simulink model "CusakisME4901"  (R2013a)
settings: Solver=ode3  StartTime=0.0  StopTime=inf  FixedStep=0.01  RelTol=1e-3
InitFcn:
  | start_EEVSCube2
  | 
  | %links masses
  | 
  | m=20;%Kg
  | 
  | l=1;%meter
  | 
  | w=0.08;
  | 
  | I=(1/12)*m*(l^2); %moment of inertia
  | 
  | %estimation error
  | 
  | mn=20+m*0.05;
  | In=I+I*0.1;
  | 
  | %controls
  | 
  | a=0.7; %singularity positive gain
  | 
  | %Chaser
  | mb=1000;%kg
  | lc=2;%meters
  | lb=lc/2;%meter distance 1joint to CM
  | Ib=(1/12)*mb*(lc^2+lc^2);
  | 
  | %Target
  | 
  | mt=750;%kg target mass
  | lt=1;%meter  side lenght
  | It=(1/6)*(lt^2)*mt;
  | 
  | %Target Initial Conitions
  | 
  | x_t=2;
  | y_t=2;
  | theta_t=0.7853;
  | 
  | Init_t=[x_t;y_t;theta_t;0;0;0];
  | Iinv=pinv(eye(3)*It);
StopFcn:
  | figure(1)
  | subplot(2,1,1)
  | hold on
  | plot(time,kinetic,'g')
  | grid on
  | title('Kinetic Energy vs Time')
  | xlabel('Time')
  | ylabel('Kinetic Energy')
  | hold off
  | 
  | subplot(2,1,2)
  | hold on
  | plot(time,power,'g')
  | grid on
  | title('Power Consumption vs Time')
  | xlabel('Time')
  | ylabel('Power')
  | hold off
  | 
  | chasermapping=[-1,1;-1,-1;1,-1;1,1;-1,1];
  | targetmapping=[1.293,2;2,2.707;2.707,2;2,1.293;1.293,2];
  | 
  | figure(3)
  | hold on
  | plot(EEstate(:,1),EEstate(:,2),'g')
  | plot(targetmapping(:,1),targetmapping(:,2),'r')
  | plot(chasermapping(:,1),chasermapping(:,2),'b')
  | grid on
  | title('End Effector Path')
  | xlabel('X Axis (m)')
  | ylabel('Y Axis (m)')
  | hold off
  | 
  | 
  | figure(4)
  | subplot(2,1,1)
  | hold on
  | plot(time,qqd(:,1),'g')
  | plot(time,qqd(:,2),'r')
  | plot(time,qqd(:,3),'b')
  | grid on
  | title('Theta vs Time')
  | xlabel('Time (sec)')
  | ylabel('Theta (rad)')
  | legend( 'Theta1 ' , ' Theta2 ' , ' Theta3')
  | hold off
  | 
  | subplot(2,1,2)
  | hold on
  | plot(time,qqd(:,4),'g')
  | plot(time,qqd(:,5),'r')
  | plot(time,qqd(:,6),'b')
  | grid on
  | legend( 'Omega1 ' , ' Omega2 ', ' Omega3 ' )
  | title('Omega vs Time')
  | xlabel('Time (sec)')
  | ylabel('Omega (rad/s)')
values from neighbouring files (symbols this model uses):
  mesh_A = [mesh_A1 ... (first row only)    [start_EEVSCube2.m]
  mesh_B = [mesh_B1 ... (first row only)    [start_EEVSCube2.m]
undefined symbols (not defined in the file or in its folder): serial
libraries: instrumentlib x5, simulink x3, vrlib x2, dspinverses x1, aerolibanimutils x1
(part 2 of 4)

== matlab function CusakisME4901/Dynamics Block/C Matrix ==
  data: qqd input; C output; mn parameter; l parameter; q_dot output
function [C,q_dot] = fcn(qqd,mn,l)
q=[qqd(7); qqd(8); qqd(9)];
q_dot=[qqd(4); qqd(5); qqd(6)];
C=[                                                                                                                                                                                                                                                                                                                                                                                                                                                                                                                                                  (mn*abs(l)^2*(2*sin(conj(q(1))) + sin(conj(q(1)) + conj(q(2)) + conj(q(3))) + 2*sin(conj(q(1)) + conj(q(2))))*(cos(q(1) + q(2) + q(3))*(q_dot(1) + q_dot(2) + q_dot(3)) + 2*cos(q(1) + q(2))*(q_dot(1) + q_dot(2)) + 2*q_dot(1)*cos(q(1))))/8 - (mn*abs(l)^2*(2*cos(conj(q(1))) + cos(conj(q(1)) + conj(q(2)) + conj(q(3))) + 2*cos(conj(q(1)) + conj(q(2))))*(sin(q(1) + q(2) + q(3))*(q_dot(1) + q_dot(2) + q_dot(3)) + 2*sin(q(1) + q(2))*(q_dot(1) + q_dot(2)) + 2*q_dot(1)*sin(q(1))))/8 + (mn*abs(l)^2*(cos(q(1) + q(2))*(q_dot(1) + q_dot(2)) + 2*q_dot(1)*cos(q(1)))*(2*sin(conj(q(1))) + sin(conj(q(1)) + conj(q(2)))))/8 - (mn*abs(l)^2*(2*cos(conj(q(1))) + cos(conj(q(1)) + conj(q(2))))*(sin(q(1) + q(2))*(q_dot(1) + q_dot(2)) + 2*q_dot(1)*sin(q(1))))/8 - (mn*abs(l)^2*(cos(q(1) + q(2)) + 2*cos(q(1)))*(2*sin(conj(q(1)))*conj(q_dot(1)) + sin(conj(q(1)) + conj(q(2)))*(conj(q_dot(1)) + conj(q_dot(2)))))/8 + (mn*abs(l)^2*(sin(q(1) + q(2)) + 2*sin(q(1)))*(2*cos(conj(q(1)))*conj(q_dot(1)) + cos(conj(q(1)) + conj(q(2)))*(conj(q_dot(1)) + conj(q_dot(2)))))/8 + (mn*abs(l)^2*(2*cos(conj(q(1)))*conj(q_dot(1)) + cos(conj(q(1)) + conj(q(2)) + conj(q(3)))*(conj(q_dot(1)) + conj(q_dot(2)) + conj(q_dot(3))) + 2*cos(conj(q(1)) + conj(q(2)))*(conj(q_dot(1)) + conj(q_dot(2))))*(sin(q(1) + q(2) + q(3)) + 2*sin(q(1) + q(2)) + 2*sin(q(1))))/8 - (mn*abs(l)^2*(2*sin(conj(q(1)))*conj(q_dot(1)) + sin(conj(q(1)) + conj(q(2)) + conj(q(3)))*(conj(q_dot(1)) + conj(q_dot(2)) + conj(q_dot(3))) + 2*sin(conj(q(1)) + conj(q(2)))*(conj(q_dot(1)) + conj(q_dot(2))))*(cos(q(1) + q(2) + q(3)) + 2*cos(q(1) + q(2)) + 2*cos(q(1))))/8 - (mn*q_dot(1)*cos(conj(q(1)))*abs(l)^2*sin(q(1)))/8 + (mn*q_dot(1)*sin(conj(q(1)))*abs(l)^2*cos(q(1)))/8 + (mn*cos(conj(q(1)))*abs(l)^2*conj(q_dot(1))*sin(q(1)))/8 - (mn*sin(conj(q(1)))*abs(l)^2*cos(q(1))*conj(q_dot(1)))/8,                                                                                                                                                                                                                                     (mn*sin(conj(q(1)) - q(2) - q(3) - q(1))*abs(l)^2)/2 + (3*mn*sin(conj(q(1)) - q(2) - q(1))*abs(l)^2)/4 + (mn*abs(l)^2*sin(conj(q(1)) - q(2) - q(3) - q(1) + conj(q(2)))*(q_dot(1) + q_dot(2) + q_dot(3) - conj(q_dot(1)) - conj(q_dot(2))))/4 + (mn*sin(conj(q(1)) - q(2) - q(3) - q(1) + conj(q(2)) + conj(q(3)))*abs(l)^2*(q_dot(1) + q_dot(2) + q_dot(3) - conj(q_dot(1)) - conj(q_dot(2)) - conj(q_dot(3))))/8 - (mn*sin(q(1) + q(2))*abs(l)^2*(2*cos(conj(q(1))) + cos(conj(q(1)) + conj(q(2)))))/8 + (mn*cos(q(1) + q(2))*abs(l)^2*(2*sin(conj(q(1))) + sin(conj(q(1)) + conj(q(2)))))/8 - (mn*abs(l)^2*(sin(conj(q(1)) + conj(q(2)) + conj(q(3))) + 2*sin(conj(q(1)) + conj(q(2))))*(cos(q(1) + q(2) + q(3)) + 2*cos(q(1) + q(2)) + 2*cos(q(1))))/8 + (mn*abs(l)^2*(cos(conj(q(1)) + conj(q(2)) + conj(q(3))) + 2*cos(conj(q(1)) + conj(q(2))))*(sin(q(1) + q(2) + q(3)) + 2*sin(q(1) + q(2)) + 2*sin(q(1))))/8 - (mn*abs(l)^2*sin(conj(q(1)) - q(2) - q(1) + conj(q(2)) + conj(q(3)))*(conj(q_dot(1)) - q_dot(2) - q_dot(1) + conj(q_dot(2)) + conj(q_dot(3))))/4 - (mn*abs(l)^2*(sin(q(1) + q(2) + q(3)) + 2*sin(q(1) + q(2)))*(2*cos(conj(q(1))) + cos(conj(q(1)) + conj(q(2)) + conj(q(3))) + 2*cos(conj(q(1)) + conj(q(2)))))/8 + (mn*abs(l)^2*(cos(q(1) + q(2) + q(3)) + 2*cos(q(1) + q(2)))*(2*sin(conj(q(1))) + sin(conj(q(1)) + conj(q(2)) + conj(q(3))) + 2*sin(conj(q(1)) + conj(q(2)))))/8 - (mn*sin(conj(q(1)) + conj(q(2)))*abs(l)^2*(cos(q(1) + q(2)) + 2*cos(q(1))))/8 + (3*mn*sin(conj(q(1)) - q(2) - q(1))*abs(l)^2*(q_dot(1) + q_dot(2) - conj(q_dot(1))))/4 + (mn*cos(conj(q(1)) + conj(q(2)))*abs(l)^2*(sin(q(1) + q(2)) + 2*sin(q(1))))/8 + (5*mn*sin(conj(q(1)) - q(2) - q(1) + conj(q(2)))*abs(l)^2*(q_dot(1) + q_dot(2) - conj(q_dot(1)) - conj(q_dot(2))))/8 + (mn*sin(conj(q(1)) - q(2) - q(3) - q(1))*abs(l)^2*(q_dot(1) + q_dot(2) + q_dot(3) - conj(q_dot(1))))/4, (mn*sin(conj(q(1)) - q(2) - q(3) - q(1))*abs(l)^2)/4 + (mn*abs(l)^2*(2*sin(conj(q(1)) - q(2) - q(3) - q(1)) + 2*sin(conj(q(1)) - q(2) - q(3) - q(1) + conj(q(2)))))/8 + (mn*abs(l)^2*(2*sin(conj(q(1)) - q(2) - q(3) - q(1))*(q_dot(1) + q_dot(2) + q_dot(3) - conj(q_dot(1))) + 2*sin(conj(q(1)) - q(2) - q(3) - q(1) + conj(q(2)))*(q_dot(1) + q_dot(2) + q_dot(3) - conj(q_dot(1)) - conj(q_dot(2))) + sin(conj(q(1)) - q(2) - q(3) - q(1) + conj(q(2)) + conj(q(3)))*(q_dot(1) + q_dot(2) + q_dot(3) - conj(q_dot(1)) - conj(q_dot(2)) - conj(q_dot(3)))))/8 + (mn*abs(l)^2*sin(conj(q(1)) - q(2) - q(3) - q(1) + conj(q(2))))/4 - (mn*abs(l)^2*sin(conj(q(1)) - q(2) - q(1) + conj(q(2)) + conj(q(3))))/4 + (mn*cos(conj(q(1)) + conj(q(2)) + conj(q(3)))*abs(l)^2*(sin(q(1) + q(2) + q(3)) + 2*sin(q(1) + q(2)) + 2*sin(q(1))))/8 - (mn*sin(q(1) + q(2) + q(3))*abs(l)^2*(2*cos(conj(q(1))) + cos(conj(q(1)) + conj(q(2)) + conj(q(3))) + 2*cos(conj(q(1)) + conj(q(2)))))/8 + (mn*cos(q(1) + q(2) + q(3))*abs(l)^2*(2*sin(conj(q(1))) + sin(conj(q(1)) + conj(q(2)) + conj(q(3))) + 2*sin(conj(q(1)) + conj(q(2)))))/8 - (mn*sin(conj(q(1)) + conj(q(2)) + conj(q(3)))*abs(l)^2*(cos(q(1) + q(2) + q(3)) + 2*cos(q(1) + q(2)) + 2*cos(q(1))))/8;
 (mn*sin(conj(q(1)) - q(2) - q(3) - q(1))*abs(l)^2)/2 + (3*mn*sin(conj(q(1)) - q(2) - q(1))*abs(l)^2)/4 - (mn*abs(l)^2*(cos(conj(q(1)) + conj(q(2)) + conj(q(3))) + 2*cos(conj(q(1)) + conj(q(2))))*(sin(q(1) + q(2) + q(3))*(q_dot(1) + q_dot(2) + q_dot(3)) + 2*sin(q(1) + q(2))*(q_dot(1) + q_dot(2)) + 2*q_dot(1)*sin(q(1))))/8 - (mn*sin(q(1) + q(2))*abs(l)^2*(2*cos(conj(q(1))) + cos(conj(q(1)) + conj(q(2)))))/8 + (mn*cos(q(1) + q(2))*abs(l)^2*(2*sin(conj(q(1))) + sin(conj(q(1)) + conj(q(2)))))/8 - (mn*abs(l)^2*(sin(conj(q(1)) + conj(q(2)) + conj(q(3))) + 2*sin(conj(q(1)) + conj(q(2))))*(cos(q(1) + q(2) + q(3)) + 2*cos(q(1) + q(2)) + 2*cos(q(1))))/8 + (mn*abs(l)^2*(cos(conj(q(1)) + conj(q(2)) + conj(q(3))) + 2*cos(conj(q(1)) + conj(q(2))))*(sin(q(1) + q(2) + q(3)) + 2*sin(q(1) + q(2)) + 2*sin(q(1))))/8 - (mn*abs(l)^2*(sin(conj(q(1)) + conj(q(2)) + conj(q(3)))*(conj(q_dot(1)) + conj(q_dot(2)) + conj(q_dot(3))) + 2*sin(conj(q(1)) + conj(q(2)))*(conj(q_dot(1)) + conj(q_dot(2))))*(cos(q(1) + q(2) + q(3)) + 2*cos(q(1) + q(2)) + 2*cos(q(1))))/8 + (mn*abs(l)^2*(cos(conj(q(1)) + conj(q(2)) + conj(q(3)))*(conj(q_dot(1)) + conj(q_dot(2)) + conj(q_dot(3))) + 2*cos(conj(q(1)) + conj(q(2)))*(conj(q_dot(1)) + conj(q_dot(2))))*(sin(q(1) + q(2) + q(3)) + 2*sin(q(1) + q(2)) + 2*sin(q(1))))/8 - (mn*abs(l)^2*(sin(q(1) + q(2) + q(3)) + 2*sin(q(1) + q(2)))*(2*cos(conj(q(1))) + cos(conj(q(1)) + conj(q(2)) + conj(q(3))) + 2*cos(conj(q(1)) + conj(q(2)))))/8 + (mn*abs(l)^2*(cos(q(1) + q(2) + q(3)) + 2*cos(q(1) + q(2)))*(2*sin(conj(q(1))) + sin(conj(q(1)) + conj(q(2)) + conj(q(3))) + 2*sin(conj(q(1)) + conj(q(2)))))/8 - (mn*sin(conj(q(1)) + conj(q(2)))*abs(l)^2*(cos(q(1) + q(2)) + 2*cos(q(1))))/8 + (mn*cos(conj(q(1)) + conj(q(2)))*abs(l)^2*(sin(q(1) + q(2)) + 2*sin(q(1))))/8 + (mn*sin(conj(q(1)) + conj(q(2)))*abs(l)^2*(cos(q(1) + q(2))*(q_dot(1) + q_dot(2)) + 2*q_dot(1)*cos(q(1))))/8 - (mn*cos(conj(q(1)) + conj(q(2)))*abs(l)^2*(sin(q(1) + q(2))*(q_dot(1) + q_dot(2)) + 2*q_dot(1)*sin(q(1))))/8 + (mn*abs(l)^2*(sin(conj(q(1)) + conj(q(2)) + conj(q(3))) + 2*sin(conj(q(1)) + conj(q(2))))*(cos(q(1) + q(2) + q(3))*(q_dot(1) + q_dot(2) + q_dot(3)) + 2*cos(q(1) + q(2))*(q_dot(1) + q_dot(2)) + 2*q_dot(1)*cos(q(1))))/8 - (mn*sin(conj(q(1)) + conj(q(2)))*abs(l)^2*(conj(q_dot(1)) + conj(q_dot(2)))*(cos(q(1) + q(2)) + 2*cos(q(1))))/8 + (mn*cos(conj(q(1)) + conj(q(2)))*abs(l)^2*(conj(q_dot(1)) + conj(q_dot(2)))*(sin(q(1) + q(2)) + 2*sin(q(1))))/8, (mn*sin(conj(q(1)) + conj(q(2)))*cos(q(1) + q(2))*abs(l)^2)/4 - (mn*cos(conj(q(1)) + conj(q(2)))*sin(q(1) + q(2))*abs(l)^2)/4 - (mn*abs(l)^2*(sin(conj(q(1)) + conj(q(2)) + conj(q(3))) + 2*sin(conj(q(1)) + conj(q(2))))*(cos(q(1) + q(2) + q(3)) + 2*cos(q(1) + q(2)) + 2*cos(q(1))))/4 + (mn*abs(l)^2*(cos(conj(q(1)) + conj(q(2)) + conj(q(3))) + 2*cos(conj(q(1)) + conj(q(2))))*(sin(q(1) + q(2) + q(3)) + 2*sin(q(1) + q(2)) + 2*sin(q(1))))/4 - (mn*abs(l)^2*(cos(q(1) + q(2) + q(3)) + 2*cos(q(1) + q(2)))*(sin(conj(q(1)) + conj(q(2)) + conj(q(3)))*(conj(q_dot(1)) + conj(q_dot(2)) + conj(q_dot(3))) + 2*sin(conj(q(1)) + conj(q(2)))*(conj(q_dot(1)) + conj(q_dot(2)))))/8 + (mn*abs(l)^2*(sin(q(1) + q(2) + q(3)) + 2*sin(q(1) + q(2)))*(cos(conj(q(1)) + conj(q(2)) + conj(q(3)))*(conj(q_dot(1)) + conj(q_dot(2)) + conj(q_dot(3))) + 2*cos(conj(q(1)) + conj(q(2)))*(conj(q_dot(1)) + conj(q_dot(2)))))/8 - (mn*abs(l)^2*(cos(conj(q(1)) + conj(q(2)) + conj(q(3))) + 2*cos(conj(q(1)) + conj(q(2))))*(sin(q(1) + q(2) + q(3))*(q_dot(1) + q_dot(2) + q_dot(3)) + 2*sin(q(1) + q(2))*(q_dot(1) + q_dot(2))))/8 + (mn*abs(l)^2*(sin(conj(q(1)) + conj(q(2)) + conj(q(3))) + 2*sin(conj(q(1)) + conj(q(2))))*(cos(q(1) + q(2) + q(3))*(q_dot(1) + q_dot(2) + q_dot(3)) + 2*cos(q(1) + q(2))*(q_dot(1) + q_dot(2))))/8 - (mn*sin(conj(q(1)) + conj(q(2)))*abs(l)^2*(cos(q(1) + q(2)) + 2*cos(q(1))))/4 + (mn*cos(conj(q(1)) + conj(q(2)))*abs(l)^2*(sin(q(1) + q(2)) + 2*sin(q(1))))/4 - (mn*abs(l)^2*(cos(conj(q(1)) + conj(q(2)) + conj(q(3))) + 2*cos(conj(q(1)) + conj(q(2))))*(sin(q(1) + q(2) + q(3)) + 2*sin(q(1) + q(2))))/4 + (mn*abs(l)^2*(cos(q(1) + q(2) + q(3)) + 2*cos(q(1) + q(2)))*(sin(conj(q(1)) + conj(q(2)) + conj(q(3))) + 2*sin(conj(q(1)) + conj(q(2)))))/4 + (mn*cos(conj(q(1)) + conj(q(2)))*sin(q(1) + q(2))*abs(l)^2*(conj(q_dot(1)) + conj(q_dot(2))))/8 - (mn*sin(conj(q(1)) + conj(q(2)))*cos(q(1) + q(2))*abs(l)^2*(conj(q_dot(1)) + conj(q_dot(2))))/8 - (mn*cos(conj(q(1)) + conj(q(2)))*sin(q(1) + q(2))*abs(l)^2*(q_dot(1) + q_dot(2)))/8 + (mn*sin(conj(q(1)) + conj(q(2)))*cos(q(1) + q(2))*abs(l)^2*(q_dot(1) + q_dot(2)))/8,                                                                                                                                                                                                                                                                                                                       (mn*abs(l)^2*(2*sin(conj(q(1)) - q(2) - q(3) - q(1) + conj(q(2)))*(q_dot(1) + q_dot(2) + q_dot(3) - conj(q_dot(1)) - conj(q_dot(2))) + sin(conj(q(1)) - q(2) - q(3) - q(1) + conj(q(2)) + conj(q(3)))*(q_dot(1) + q_dot(2) + q_dot(3) - conj(q_dot(1)) - conj(q_dot(2)) - conj(q_dot(3)))))/8 + (mn*abs(l)^2*sin(conj(q(1)) - q(2) - q(3) - q(1) + conj(q(2))))/4 + (mn*cos(conj(q(1)) + conj(q(2)) + conj(q(3)))*abs(l)^2*(sin(q(1) + q(2) + q(3)) + 2*sin(q(1) + q(2)) + 2*sin(q(1))))/4 - (mn*sin(q(1) + q(2) + q(3))*abs(l)^2*(cos(conj(q(1)) + conj(q(2)) + conj(q(3))) + 2*cos(conj(q(1)) + conj(q(2)))))/4 + (mn*cos(q(1) + q(2) + q(3))*abs(l)^2*(sin(conj(q(1)) + conj(q(2)) + conj(q(3))) + 2*sin(conj(q(1)) + conj(q(2)))))/4 - (mn*sin(conj(q(1)) + conj(q(2)) + conj(q(3)))*abs(l)^2*(cos(q(1) + q(2) + q(3)) + 2*cos(q(1) + q(2)) + 2*cos(q(1))))/4;
                                                                                                                                                                                                                                                                                                                                                                                                                                                                                                                                                                                                                                                                                                                                                                                                      (mn*sin(conj(q(1)) - q(2) - q(3) - q(1))*abs(l)^2)/4 + (mn*abs(l)^2*(2*sin(conj(q(1)) - q(2) - q(3) - q(1)) + 2*sin(conj(q(1)) - q(2) - q(3) - q(1) + conj(q(2)))))/8 + (mn*abs(l)^2*sin(conj(q(1)) - q(2) - q(3) - q(1) + conj(q(2))))/4 - (mn*abs(l)^2*sin(conj(q(1)) - q(2) - q(1) + conj(q(2)) + conj(q(3))))/4 + (mn*cos(conj(q(1)) + conj(q(2)) + conj(q(3)))*abs(l)^2*(sin(q(1) + q(2) + q(3)) + 2*sin(q(1) + q(2)) + 2*sin(q(1))))/8 - (mn*sin(q(1) + q(2) + q(3))*abs(l)^2*(2*cos(conj(q(1))) + cos(conj(q(1)) + conj(q(2)) + conj(q(3))) + 2*cos(conj(q(1)) + conj(q(2)))))/8 + (mn*cos(q(1) + q(2) + q(3))*abs(l)^2*(2*sin(conj(q(1))) + sin(conj(q(1)) + conj(q(2)) + conj(q(3))) + 2*sin(conj(q(1)) + conj(q(2)))))/8 + (mn*sin(conj(q(1)) + conj(q(2)) + conj(q(3)))*abs(l)^2*(cos(q(1) + q(2) + q(3))*(q_dot(1) + q_dot(2) + q_dot(3)) + 2*cos(q(1) + q(2))*(q_dot(1) + q_dot(2)) + 2*q_dot(1)*cos(q(1))))/8 - (mn*cos(conj(q(1)) + conj(q(2)) + conj(q(3)))*abs(l)^2*(sin(q(1) + q(2) + q(3))*(q_dot(1) + q_dot(2) + q_dot(3)) + 2*sin(q(1) + q(2))*(q_dot(1) + q_dot(2)) + 2*q_dot(1)*sin(q(1))))/8 - (mn*sin(conj(q(1)) + conj(q(2)) + conj(q(3)))*abs(l)^2*(cos(q(1) + q(2) + q(3)) + 2*cos(q(1) + q(2)) + 2*cos(q(1))))/8 - (mn*sin(conj(q(1)) + conj(q(2)) + conj(q(3)))*abs(l)^2*(cos(q(1) + q(2) + q(3)) + 2*cos(q(1) + q(2)) + 2*cos(q(1)))*(conj(q_dot(1)) + conj(q_dot(2)) + conj(q_dot(3))))/8 + (mn*cos(conj(q(1)) + conj(q(2)) + conj(q(3)))*abs(l)^2*(sin(q(1) + q(2) + q(3)) + 2*sin(q(1) + q(2)) + 2*sin(q(1)))*(conj(q_dot(1)) + conj(q_dot(2)) + conj(q_dot(3))))/8,                                                                                                                                                                                                                                                                                                                                                                                                                                                                                                                                                                                                                                                                                                                                                                                                            (mn*abs(l)^2*sin(conj(q(1)) - q(2) - q(3) - q(1) + conj(q(2))))/4 + (mn*cos(conj(q(1)) + conj(q(2)) + conj(q(3)))*abs(l)^2*(sin(q(1) + q(2) + q(3)) + 2*sin(q(1) + q(2)) + 2*sin(q(1))))/4 + (mn*sin(conj(q(1)) + conj(q(2)) + conj(q(3)))*abs(l)^2*(cos(q(1) + q(2) + q(3))*(q_dot(1) + q_dot(2) + q_dot(3)) + 2*cos(q(1) + q(2))*(q_dot(1) + q_dot(2))))/8 - (mn*cos(conj(q(1)) + conj(q(2)) + conj(q(3)))*abs(l)^2*(sin(q(1) + q(2) + q(3))*(q_dot(1) + q_dot(2) + q_dot(3)) + 2*sin(q(1) + q(2))*(q_dot(1) + q_dot(2))))/8 - (mn*sin(q(1) + q(2) + q(3))*abs(l)^2*(cos(conj(q(1)) + conj(q(2)) + conj(q(3))) + 2*cos(conj(q(1)) + conj(q(2)))))/4 + (mn*cos(q(1) + q(2) + q(3))*abs(l)^2*(sin(conj(q(1)) + conj(q(2)) + conj(q(3))) + 2*sin(conj(q(1)) + conj(q(2)))))/4 - (mn*sin(conj(q(1)) + conj(q(2)) + conj(q(3)))*abs(l)^2*(cos(q(1) + q(2) + q(3)) + 2*cos(q(1) + q(2)) + 2*cos(q(1))))/4 - (mn*sin(conj(q(1)) + conj(q(2)) + conj(q(3)))*abs(l)^2*(cos(q(1) + q(2) + q(3)) + 2*cos(q(1) + q(2)))*(conj(q_dot(1)) + conj(q_dot(2)) + conj(q_dot(3))))/8 + (mn*cos(conj(q(1)) + conj(q(2)) + conj(q(3)))*abs(l)^2*(sin(q(1) + q(2) + q(3)) + 2*sin(q(1) + q(2)))*(conj(q_dot(1)) + conj(q_dot(2)) + conj(q_dot(3))))/8,                                                                                                                                                                                                                                                                                                                                                            (mn*sin(conj(q(1)) - q(2) - q(3) - q(1) + conj(q(2)) + conj(q(3)))*abs(l)^2*(q_dot(1) + q_dot(2) + q_dot(3) - conj(q_dot(1)) - conj(q_dot(2)) - conj(q_dot(3))))/8 + (mn*cos(conj(q(1)) + conj(q(2)) + conj(q(3)))*abs(l)^2*(sin(q(1) + q(2) + q(3)) + 2*sin(q(1) + q(2)) + 2*sin(q(1))))/4 + (mn*cos(q(1) + q(2) + q(3))*sin(conj(q(1)) + conj(q(2)) + conj(q(3)))*abs(l)^2)/2 - (mn*sin(q(1) + q(2) + q(3))*cos(conj(q(1)) + conj(q(2)) + conj(q(3)))*abs(l)^2)/2 - (mn*sin(conj(q(1)) + conj(q(2)) + conj(q(3)))*abs(l)^2*(cos(q(1) + q(2) + q(3)) + 2*cos(q(1) + q(2))))/4 + (mn*cos(conj(q(1)) + conj(q(2)) + conj(q(3)))*abs(l)^2*(sin(q(1) + q(2) + q(3)) + 2*sin(q(1) + q(2))))/4 - (mn*sin(conj(q(1)) + conj(q(2)) + conj(q(3)))*abs(l)^2*(cos(q(1) + q(2) + q(3)) + 2*cos(q(1) + q(2)) + 2*cos(q(1))))/4];

== matlab function CusakisME4901/Dynamics Block/G Matrix (set to zero) ==
  data: qqd input; G output; l parameter; m parameter
function G = fcn(qqd,l,m)

q=[qqd(7) qqd(8) qqd(9)];

g=[0 9.81 0]; %gravity acceleration along y


Jp1=[-(l/2)*sin(q(1)) 0 0; (l/2)*cos(q(1)) 0 0; 0 0 0];
Jo1=[0 0 0; 0 0 0; 1 0 0];

Jp2=[-l*sin(q(1))-(l/2)*sin(q(1)+q(2)) -(l/2)*sin(q(1)+q(2)) 0 ;    l*cos(q(1))+(l/2)*cos(q(1)+q(2)) (l/2)*cos(q(1)+q(2)) 0; 0 0 0];
Jo2=[0 0 0; 0 0 0; 1 1 0];

Jp3=[-l*sin(q(1))-l*sin(q(1)+q(2))-(l/2)*sin(q(1)+q(2)+q(3)) -l*sin(q(1)+q(2))-(l/2)*sin(q(1)+q(2)+q(3)) -(l/2)*sin(q(1)+q(2)+q(3)); l*cos(q(1))+(l)*cos(q(1)+q(2))+(l/2)*cos(q(1)+q(2)+q(3)) l*cos(q(1)+q(2))+(l/2)*cos(q(1)+q(2)+q(3)) (l/2)*cos(q(1)+q(2)+q(3)); 0 0 0];
Jo3=[0 0 0; 0 0 0; 1 1 1];

G1=m*(g)*Jp1+m*(g)*Jp2+m*(g)*Jp3;

%G=G1.';

G=[0;0;0];

== matlab function CusakisME4901/Torque Control/C Matrix ==
  data: qqd input; C output; m parameter; l parameter; q_dot output
function [C,q_dot] = fcn(qqd,m,l)
q=[qqd(7); qqd(8); qqd(9)];
q_dot=[qqd(4); qqd(5); qqd(6)];
C=[                                                                                                                                                                                                                                                                                                                                                                                                                                                                                                                                                  (m*abs(l)^2*(2*sin(conj(q(1))) + sin(conj(q(1)) + conj(q(2)) + conj(q(3))) + 2*sin(conj(q(1)) + conj(q(2))))*(cos(q(1) + q(2) + q(3))*(q_dot(1) + q_dot(2) + q_dot(3)) + 2*cos(q(1) + q(2))*(q_dot(1) + q_dot(2)) + 2*q_dot(1)*cos(q(1))))/8 - (m*abs(l)^2*(2*cos(conj(q(1))) + cos(conj(q(1)) + conj(q(2)) + conj(q(3))) + 2*cos(conj(q(1)) + conj(q(2))))*(sin(q(1) + q(2) + q(3))*(q_dot(1) + q_dot(2) + q_dot(3)) + 2*sin(q(1) + q(2))*(q_dot(1) + q_dot(2)) + 2*q_dot(1)*sin(q(1))))/8 + (m*abs(l)^2*(cos(q(1) + q(2))*(q_dot(1) + q_dot(2)) + 2*q_dot(1)*cos(q(1)))*(2*sin(conj(q(1))) + sin(conj(q(1)) + conj(q(2)))))/8 - (m*abs(l)^2*(2*cos(conj(q(1))) + cos(conj(q(1)) + conj(q(2))))*(sin(q(1) + q(2))*(q_dot(1) + q_dot(2)) + 2*q_dot(1)*sin(q(1))))/8 - (m*abs(l)^2*(cos(q(1) + q(2)) + 2*cos(q(1)))*(2*sin(conj(q(1)))*conj(q_dot(1)) + sin(conj(q(1)) + conj(q(2)))*(conj(q_dot(1)) + conj(q_dot(2)))))/8 + (m*abs(l)^2*(sin(q(1) + q(2)) + 2*sin(q(1)))*(2*cos(conj(q(1)))*conj(q_dot(1)) + cos(conj(q(1)) + conj(q(2)))*(conj(q_dot(1)) + conj(q_dot(2)))))/8 + (m*abs(l)^2*(2*cos(conj(q(1)))*conj(q_dot(1)) + cos(conj(q(1)) + conj(q(2)) + conj(q(3)))*(conj(q_dot(1)) + conj(q_dot(2)) + conj(q_dot(3))) + 2*cos(conj(q(1)) + conj(q(2)))*(conj(q_dot(1)) + conj(q_dot(2))))*(sin(q(1) + q(2) + q(3)) + 2*sin(q(1) + q(2)) + 2*sin(q(1))))/8 - (m*abs(l)^2*(2*sin(conj(q(1)))*conj(q_dot(1)) + sin(conj(q(1)) + conj(q(2)) + conj(q(3)))*(conj(q_dot(1)) + conj(q_dot(2)) + conj(q_dot(3))) + 2*sin(conj(q(1)) + conj(q(2)))*(conj(q_dot(1)) + conj(q_dot(2))))*(cos(q(1) + q(2) + q(3)) + 2*cos(q(1) + q(2)) + 2*cos(q(1))))/8 - (m*q_dot(1)*cos(conj(q(1)))*abs(l)^2*sin(q(1)))/8 + (m*q_dot(1)*sin(conj(q(1)))*abs(l)^2*cos(q(1)))/8 + (m*cos(conj(q(1)))*abs(l)^2*conj(q_dot(1))*sin(q(1)))/8 - (m*sin(conj(q(1)))*abs(l)^2*cos(q(1))*conj(q_dot(1)))/8,                                                                                                                                                                                                                                     (m*sin(conj(q(1)) - q(2) - q(3) - q(1))*abs(l)^2)/2 + (3*m*sin(conj(q(1)) - q(2) - q(1))*abs(l)^2)/4 + (m*abs(l)^2*sin(conj(q(1)) - q(2) - q(3) - q(1) + conj(q(2)))*(q_dot(1) + q_dot(2) + q_dot(3) - conj(q_dot(1)) - conj(q_dot(2))))/4 + (m*sin(conj(q(1)) - q(2) - q(3) - q(1) + conj(q(2)) + conj(q(3)))*abs(l)^2*(q_dot(1) + q_dot(2) + q_dot(3) - conj(q_dot(1)) - conj(q_dot(2)) - conj(q_dot(3))))/8 - (m*sin(q(1) + q(2))*abs(l)^2*(2*cos(conj(q(1))) + cos(conj(q(1)) + conj(q(2)))))/8 + (m*cos(q(1) + q(2))*abs(l)^2*(2*sin(conj(q(1))) + sin(conj(q(1)) + conj(q(2)))))/8 - (m*abs(l)^2*(sin(conj(q(1)) + conj(q(2)) + conj(q(3))) + 2*sin(conj(q(1)) + conj(q(2))))*(cos(q(1) + q(2) + q(3)) + 2*cos(q(1) + q(2)) + 2*cos(q(1))))/8 + (m*abs(l)^2*(cos(conj(q(1)) + conj(q(2)) + conj(q(3))) + 2*cos(conj(q(1)) + conj(q(2))))*(sin(q(1) + q(2) + q(3)) + 2*sin(q(1) + q(2)) + 2*sin(q(1))))/8 - (m*abs(l)^2*sin(conj(q(1)) - q(2) - q(1) + conj(q(2)) + conj(q(3)))*(conj(q_dot(1)) - q_dot(2) - q_dot(1) + conj(q_dot(2)) + conj(q_dot(3))))/4 - (m*abs(l)^2*(sin(q(1) + q(2) + q(3)) + 2*sin(q(1) + q(2)))*(2*cos(conj(q(1))) + cos(conj(q(1)) + conj(q(2)) + conj(q(3))) + 2*cos(conj(q(1)) + conj(q(2)))))/8 + (m*abs(l)^2*(cos(q(1) + q(2) + q(3)) + 2*cos(q(1) + q(2)))*(2*sin(conj(q(1))) + sin(conj(q(1)) + conj(q(2)) + conj(q(3))) + 2*sin(conj(q(1)) + conj(q(2)))))/8 - (m*sin(conj(q(1)) + conj(q(2)))*abs(l)^2*(cos(q(1) + q(2)) + 2*cos(q(1))))/8 + (3*m*sin(conj(q(1)) - q(2) - q(1))*abs(l)^2*(q_dot(1) + q_dot(2) - conj(q_dot(1))))/4 + (m*cos(conj(q(1)) + conj(q(2)))*abs(l)^2*(sin(q(1) + q(2)) + 2*sin(q(1))))/8 + (5*m*sin(conj(q(1)) - q(2) - q(1) + conj(q(2)))*abs(l)^2*(q_dot(1) + q_dot(2) - conj(q_dot(1)) - conj(q_dot(2))))/8 + (m*sin(conj(q(1)) - q(2) - q(3) - q(1))*abs(l)^2*(q_dot(1) + q_dot(2) + q_dot(3) - conj(q_dot(1))))/4, (m*sin(conj(q(1)) - q(2) - q(3) - q(1))*abs(l)^2)/4 + (m*abs(l)^2*(2*sin(conj(q(1)) - q(2) - q(3) - q(1)) + 2*sin(conj(q(1)) - q(2) - q(3) - q(1) + conj(q(2)))))/8 + (m*abs(l)^2*(2*sin(conj(q(1)) - q(2) - q(3) - q(1))*(q_dot(1) + q_dot(2) + q_dot(3) - conj(q_dot(1))) + 2*sin(conj(q(1)) - q(2) - q(3) - q(1) + conj(q(2)))*(q_dot(1) + q_dot(2) + q_dot(3) - conj(q_dot(1)) - conj(q_dot(2))) + sin(conj(q(1)) - q(2) - q(3) - q(1) + conj(q(2)) + conj(q(3)))*(q_dot(1) + q_dot(2) + q_dot(3) - conj(q_dot(1)) - conj(q_dot(2)) - conj(q_dot(3)))))/8 + (m*abs(l)^2*sin(conj(q(1)) - q(2) - q(3) - q(1) + conj(q(2))))/4 - (m*abs(l)^2*sin(conj(q(1)) - q(2) - q(1) + conj(q(2)) + conj(q(3))))/4 + (m*cos(conj(q(1)) + conj(q(2)) + conj(q(3)))*abs(l)^2*(sin(q(1) + q(2) + q(3)) + 2*sin(q(1) + q(2)) + 2*sin(q(1))))/8 - (m*sin(q(1) + q(2) + q(3))*abs(l)^2*(2*cos(conj(q(1))) + cos(conj(q(1)) + conj(q(2)) + conj(q(3))) + 2*cos(conj(q(1)) + conj(q(2)))))/8 + (m*cos(q(1) + q(2) + q(3))*abs(l)^2*(2*sin(conj(q(1))) + sin(conj(q(1)) + conj(q(2)) + conj(q(3))) + 2*sin(conj(q(1)) + conj(q(2)))))/8 - (m*sin(conj(q(1)) + conj(q(2)) + conj(q(3)))*abs(l)^2*(cos(q(1) + q(2) + q(3)) + 2*cos(q(1) + q(2)) + 2*cos(q(1))))/8;
 (m*sin(conj(q(1)) - q(2) - q(3) - q(1))*abs(l)^2)/2 + (3*m*sin(conj(q(1)) - q(2) - q(1))*abs(l)^2)/4 - (m*abs(l)^2*(cos(conj(q(1)) + conj(q(2)) + conj(q(3))) + 2*cos(conj(q(1)) + conj(q(2))))*(sin(q(1) + q(2) + q(3))*(q_dot(1) + q_dot(2) + q_dot(3)) + 2*sin(q(1) + q(2))*(q_dot(1) + q_dot(2)) + 2*q_dot(1)*sin(q(1))))/8 - (m*sin(q(1) + q(2))*abs(l)^2*(2*cos(conj(q(1))) + cos(conj(q(1)) + conj(q(2)))))/8 + (m*cos(q(1) + q(2))*abs(l)^2*(2*sin(conj(q(1))) + sin(conj(q(1)) + conj(q(2)))))/8 - (m*abs(l)^2*(sin(conj(q(1)) + conj(q(2)) + conj(q(3))) + 2*sin(conj(q(1)) + conj(q(2))))*(cos(q(1) + q(2) + q(3)) + 2*cos(q(1) + q(2)) + 2*cos(q(1))))/8 + (m*abs(l)^2*(cos(conj(q(1)) + conj(q(2)) + conj(q(3))) + 2*cos(conj(q(1)) + conj(q(2))))*(sin(q(1) + q(2) + q(3)) + 2*sin(q(1) + q(2)) + 2*sin(q(1))))/8 - (m*abs(l)^2*(sin(conj(q(1)) + conj(q(2)) + conj(q(3)))*(conj(q_dot(1)) + conj(q_dot(2)) + conj(q_dot(3))) + 2*sin(conj(q(1)) + conj(q(2)))*(conj(q_dot(1)) + conj(q_dot(2))))*(cos(q(1) + q(2) + q(3)) + 2*cos(q(1) + q(2)) + 2*cos(q(1))))/8 + (m*abs(l)^2*(cos(conj(q(1)) + conj(q(2)) + conj(q(3)))*(conj(q_dot(1)) + conj(q_dot(2)) + conj(q_dot(3))) + 2*cos(conj(q(1)) + conj(q(2)))*(conj(q_dot(1)) + conj(q_dot(2))))*(sin(q(1) + q(2) + q(3)) + 2*sin(q(1) + q(2)) + 2*sin(q(1))))/8 - (m*abs(l)^2*(sin(q(1) + q(2) + q(3)) + 2*sin(q(1) + q(2)))*(2*cos(conj(q(1))) + cos(conj(q(1)) + conj(q(2)) + conj(q(3))) + 2*cos(conj(q(1)) + conj(q(2)))))/8 + (m*abs(l)^2*(cos(q(1) + q(2) + q(3)) + 2*cos(q(1) + q(2)))*(2*sin(conj(q(1))) + sin(conj(q(1)) + conj(q(2)) + conj(q(3))) + 2*sin(conj(q(1)) + conj(q(2)))))/8 - (m*sin(conj(q(1)) + conj(q(2)))*abs(l)^2*(cos(q(1) + q(2)) + 2*cos(q(1))))/8 + (m*cos(conj(q(1)) + conj(q(2)))*abs(l)^2*(sin(q(1) + q(2)) + 2*sin(q(1))))/8 + (m*sin(conj(q(1)) + conj(q(2)))*abs(l)^2*(cos(q(1) + q(2))*(q_dot(1) + q_dot(2)) + 2*q_dot(1)*cos(q(1))))/8 - (m*cos(conj(q(1)) + conj(q(2)))*abs(l)^2*(sin(q(1) + q(2))*(q_dot(1) + q_dot(2)) + 2*q_dot(1)*sin(q(1))))/8 + (m*abs(l)^2*(sin(conj(q(1)) + conj(q(2)) + conj(q(3))) + 2*sin(conj(q(1)) + conj(q(2))))*(cos(q(1) + q(2) + q(3))*(q_dot(1) + q_dot(2) + q_dot(3)) + 2*cos(q(1) + q(2))*(q_dot(1) + q_dot(2)) + 2*q_dot(1)*cos(q(1))))/8 - (m*sin(conj(q(1)) + conj(q(2)))*abs(l)^2*(conj(q_dot(1)) + conj(q_dot(2)))*(cos(q(1) + q(2)) + 2*cos(q(1))))/8 + (m*cos(conj(q(1)) + conj(q(2)))*abs(l)^2*(conj(q_dot(1)) + conj(q_dot(2)))*(sin(q(1) + q(2)) + 2*sin(q(1))))/8, (m*sin(conj(q(1)) + conj(q(2)))*cos(q(1) + q(2))*abs(l)^2)/4 - (m*cos(conj(q(1)) + conj(q(2)))*sin(q(1) + q(2))*abs(l)^2)/4 - (m*abs(l)^2*(sin(conj(q(1)) + conj(q(2)) + conj(q(3))) + 2*sin(conj(q(1)) + conj(q(2))))*(cos(q(1) + q(2) + q(3)) + 2*cos(q(1) + q(2)) + 2*cos(q(1))))/4 + (m*abs(l)^2*(cos(conj(q(1)) + conj(q(2)) + conj(q(3))) + 2*cos(conj(q(1)) + conj(q(2))))*(sin(q(1) + q(2) + q(3)) + 2*sin(q(1) + q(2)) + 2*sin(q(1))))/4 - (m*abs(l)^2*(cos(q(1) + q(2) + q(3)) + 2*cos(q(1) + q(2)))*(sin(conj(q(1)) + conj(q(2)) + conj(q(3)))*(conj(q_dot(1)) + conj(q_dot(2)) + conj(q_dot(3))) + 2*sin(conj(q(1)) + conj(q(2)))*(conj(q_dot(1)) + conj(q_dot(2)))))/8 + (m*abs(l)^2*(sin(q(1) + q(2) + q(3)) + 2*sin(q(1) + q(2)))*(cos(conj(q(1)) + conj(q(2)) + conj(q(3)))*(conj(q_dot(1)) + conj(q_dot(2)) + conj(q_dot(3))) + 2*cos(conj(q(1)) + conj(q(2)))*(conj(q_dot(1)) + conj(q_dot(2)))))/8 - (m*abs(l)^2*(cos(conj(q(1)) + conj(q(2)) + conj(q(3))) + 2*cos(conj(q(1)) + conj(q(2))))*(sin(q(1) + q(2) + q(3))*(q_dot(1) + q_dot(2) + q_dot(3)) + 2*sin(q(1) + q(2))*(q_dot(1) + q_dot(2))))/8 + (m*abs(l)^2*(sin(conj(q(1)) + conj(q(2)) + conj(q(3))) + 2*sin(conj(q(1)) + conj(q(2))))*(cos(q(1) + q(2) + q(3))*(q_dot(1) + q_dot(2) + q_dot(3)) + 2*cos(q(1) + q(2))*(q_dot(1) + q_dot(2))))/8 - (m*sin(conj(q(1)) + conj(q(2)))*abs(l)^2*(cos(q(1) + q(2)) + 2*cos(q(1))))/4 + (m*cos(conj(q(1)) + conj(q(2)))*abs(l)^2*(sin(q(1) + q(2)) + 2*sin(q(1))))/4 - (m*abs(l)^2*(cos(conj(q(1)) + conj(q(2)) + conj(q(3))) + 2*cos(conj(q(1)) + conj(q(2))))*(sin(q(1) + q(2) + q(3)) + 2*sin(q(1) + q(2))))/4 + (m*abs(l)^2*(cos(q(1) + q(2) + q(3)) + 2*cos(q(1) + q(2)))*(sin(conj(q(1)) + conj(q(2)) + conj(q(3))) + 2*sin(conj(q(1)) + conj(q(2)))))/4 + (m*cos(conj(q(1)) + conj(q(2)))*sin(q(1) + q(2))*abs(l)^2*(conj(q_dot(1)) + conj(q_dot(2))))/8 - (m*sin(conj(q(1)) + conj(q(2)))*cos(q(1) + q(2))*abs(l)^2*(conj(q_dot(1)) + conj(q_dot(2))))/8 - (m*cos(conj(q(1)) + conj(q(2)))*sin(q(1) + q(2))*abs(l)^2*(q_dot(1) + q_dot(2)))/8 + (m*sin(conj(q(1)) + conj(q(2)))*cos(q(1) + q(2))*abs(l)^2*(q_dot(1) + q_dot(2)))/8,                                                                                                                                                                                                                                                                                                                       (m*abs(l)^2*(2*sin(conj(q(1)) - q(2) - q(3) - q(1) + conj(q(2)))*(q_dot(1) + q_dot(2) + q_dot(3) - conj(q_dot(1)) - conj(q_dot(2))) + sin(conj(q(1)) - q(2) - q(3) - q(1) + conj(q(2)) + conj(q(3)))*(q_dot(1) + q_dot(2) + q_dot(3) - conj(q_dot(1)) - conj(q_dot(2)) - conj(q_dot(3)))))/8 + (m*abs(l)^2*sin(conj(q(1)) - q(2) - q(3) - q(1) + conj(q(2))))/4 + (m*cos(conj(q(1)) + conj(q(2)) + conj(q(3)))*abs(l)^2*(sin(q(1) + q(2) + q(3)) + 2*sin(q(1) + q(2)) + 2*sin(q(1))))/4 - (m*sin(q(1) + q(2) + q(3))*abs(l)^2*(cos(conj(q(1)) + conj(q(2)) + conj(q(3))) + 2*cos(conj(q(1)) + conj(q(2)))))/4 + (m*cos(q(1) + q(2) + q(3))*abs(l)^2*(sin(conj(q(1)) + conj(q(2)) + conj(q(3))) + 2*sin(conj(q(1)) + conj(q(2)))))/4 - (m*sin(conj(q(1)) + conj(q(2)) + conj(q(3)))*abs(l)^2*(cos(q(1) + q(2) + q(3)) + 2*cos(q(1) + q(2)) + 2*cos(q(1))))/4;
                                                                                                                                                                                                                                                                                                                                                                                                                                                                                                                                                                                                                                                                                                                                                                                                      (m*sin(conj(q(1)) - q(2) - q(3) - q(1))*abs(l)^2)/4 + (m*abs(l)^2*(2*sin(conj(q(1)) - q(2) - q(3) - q(1)) + 2*sin(conj(q(1)) - q(2) - q(3) - q(1) + conj(q(2)))))/8 + (m*abs(l)^2*sin(conj(q(1)) - q(2) - q(3) - q(1) + conj(q(2))))/4 - (m*abs(l)^2*sin(conj(q(1)) - q(2) - q(1) + conj(q(2)) + conj(q(3))))/4 + (m*cos(conj(q(1)) + conj(q(2)) + conj(q(3)))*abs(l)^2*(sin(q(1) + q(2) + q(3)) + 2*sin(q(1) + q(2)) + 2*sin(q(1))))/8 - (m*sin(q(1) + q(2) + q(3))*abs(l)^2*(2*cos(conj(q(1))) + cos(conj(q(1)) + conj(q(2)) + conj(q(3))) + 2*cos(conj(q(1)) + conj(q(2)))))/8 + (m*cos(q(1) + q(2) + q(3))*abs(l)^2*(2*sin(conj(q(1))) + sin(conj(q(1)) + conj(q(2)) + conj(q(3))) + 2*sin(conj(q(1)) + conj(q(2)))))/8 + (m*sin(conj(q(1)) + conj(q(2)) + conj(q(3)))*abs(l)^2*(cos(q(1) + q(2) + q(3))*(q_dot(1) + q_dot(2) + q_dot(3)) + 2*cos(q(1) + q(2))*(q_dot(1) + q_dot(2)) + 2*q_dot(1)*cos(q(1))))/8 - (m*cos(conj(q(1)) + conj(q(2)) + conj(q(3)))*abs(l)^2*(sin(q(1) + q(2) + q(3))*(q_dot(1) + q_dot(2) + q_dot(3)) + 2*sin(q(1) + q(2))*(q_dot(1) + q_dot(2)) + 2*q_dot(1)*sin(q(1))))/8 - (m*sin(conj(q(1)) + conj(q(2)) + conj(q(3)))*abs(l)^2*(cos(q(1) + q(2) + q(3)) + 2*cos(q(1) + q(2)) + 2*cos(q(1))))/8 - (m*sin(conj(q(1)) + conj(q(2)) + conj(q(3)))*abs(l)^2*(cos(q(1) + q(2) + q(3)) + 2*cos(q(1) + q(2)) + 2*cos(q(1)))*(conj(q_dot(1)) + conj(q_dot(2)) + conj(q_dot(3))))/8 + (m*cos(conj(q(1)) + conj(q(2)) + conj(q(3)))*abs(l)^2*(sin(q(1) + q(2) + q(3)) + 2*sin(q(1) + q(2)) + 2*sin(q(1)))*(conj(q_dot(1)) + conj(q_dot(2)) + conj(q_dot(3))))/8,                                                                                                                                                                                                                                                                                                                                                                                                                                                                                                                                                                                                                                                                                                                                                                                                            (m*abs(l)^2*sin(conj(q(1)) - q(2) - q(3) - q(1) + conj(q(2))))/4 + (m*cos(conj(q(1)) + conj(q(2)) + conj(q(3)))*abs(l)^2*(sin(q(1) + q(2) + q(3)) + 2*sin(q(1) + q(2)) + 2*sin(q(1))))/4 + (m*sin(conj(q(1)) + conj(q(2)) + conj(q(3)))*abs(l)^2*(cos(q(1) + q(2) + q(3))*(q_dot(1) + q_dot(2) + q_dot(3)) + 2*cos(q(1) + q(2))*(q_dot(1) + q_dot(2))))/8 - (m*cos(conj(q(1)) + conj(q(2)) + conj(q(3)))*abs(l)^2*(sin(q(1) + q(2) + q(3))*(q_dot(1) + q_dot(2) + q_dot(3)) + 2*sin(q(1) + q(2))*(q_dot(1) + q_dot(2))))/8 - (m*sin(q(1) + q(2) + q(3))*abs(l)^2*(cos(conj(q(1)) + conj(q(2)) + conj(q(3))) + 2*cos(conj(q(1)) + conj(q(2)))))/4 + (m*cos(q(1) + q(2) + q(3))*abs(l)^2*(sin(conj(q(1)) + conj(q(2)) + conj(q(3))) + 2*sin(conj(q(1)) + conj(q(2)))))/4 - (m*sin(conj(q(1)) + conj(q(2)) + conj(q(3)))*abs(l)^2*(cos(q(1) + q(2) + q(3)) + 2*cos(q(1) + q(2)) + 2*cos(q(1))))/4 - (m*sin(conj(q(1)) + conj(q(2)) + conj(q(3)))*abs(l)^2*(cos(q(1) + q(2) + q(3)) + 2*cos(q(1) + q(2)))*(conj(q_dot(1)) + conj(q_dot(2)) + conj(q_dot(3))))/8 + (m*cos(conj(q(1)) + conj(q(2)) + conj(q(3)))*abs(l)^2*(sin(q(1) + q(2) + q(3)) + 2*sin(q(1) + q(2)))*(conj(q_dot(1)) + conj(q_dot(2)) + conj(q_dot(3))))/8,                                                                                                                                                                                                                                                                                                                                                            (m*sin(conj(q(1)) - q(2) - q(3) - q(1) + conj(q(2)) + conj(q(3)))*abs(l)^2*(q_dot(1) + q_dot(2) + q_dot(3) - conj(q_dot(1)) - conj(q_dot(2)) - conj(q_dot(3))))/8 + (m*cos(conj(q(1)) + conj(q(2)) + conj(q(3)))*abs(l)^2*(sin(q(1) + q(2) + q(3)) + 2*sin(q(1) + q(2)) + 2*sin(q(1))))/4 + (m*cos(q(1) + q(2) + q(3))*sin(conj(q(1)) + conj(q(2)) + conj(q(3)))*abs(l)^2)/2 - (m*sin(q(1) + q(2) + q(3))*cos(conj(q(1)) + conj(q(2)) + conj(q(3)))*abs(l)^2)/2 - (m*sin(conj(q(1)) + conj(q(2)) + conj(q(3)))*abs(l)^2*(cos(q(1) + q(2) + q(3)) + 2*cos(q(1) + q(2))))/4 + (m*cos(conj(q(1)) + conj(q(2)) + conj(q(3)))*abs(l)^2*(sin(q(1) + q(2) + q(3)) + 2*sin(q(1) + q(2))))/4 - (m*sin(conj(q(1)) + conj(q(2)) + conj(q(3)))*abs(l)^2*(cos(q(1) + q(2) + q(3)) + 2*cos(q(1) + q(2)) + 2*cos(q(1))))/4];

== matlab function CusakisME4901/Torque Control/G Matrix (set zero) ==
  data: qqd input; G output; l parameter; m parameter
function G = fcn(qqd,l,m)

q=[qqd(7); qqd(8); qqd(9)];

g=[0 9.81 0]; %gravity acceleration along y


Jp1=[-(l/2)*sin(q(1)) 0 0; (l/2)*cos(q(1)) 0 0; 0 0 0];
Jo1=[0 0 0; 0 0 0; 1 0 0];

Jp2=[-l*sin(q(1))-(l/2)*sin(q(1)+q(2)) -(l/2)*sin(q(1)+q(2)) 0 ;    l*cos(q(1))+(l/2)*cos(q(1)+q(2)) (l/2)*cos(q(1)+q(2)) 0; 0 0 0];
Jo2=[0 0 0; 0 0 0; 1 1 0];

Jp3=[-l*sin(q(1))-l*sin(q(1)+q(2))-(l/2)*sin(q(1)+q(2)+q(3)) -l*sin(q(1)+q(2))-(l/2)*sin(q(1)+q(2)+q(3)) -(l/2)*sin(q(1)+q(2)+q(3)); l*cos(q(1))+(l)*cos(q(1)+q(2))+(l/2)*cos(q(1)+q(2)+q(3)) l*cos(q(1)+q(2))+(l/2)*cos(q(1)+q(2)+q(3)) (l/2)*cos(q(1)+q(2)+q(3)); 0 0 0];
Jo3=[0 0 0; 0 0 0; 1 1 1];

G1=m*(g)*Jp1+m*(g)*Jp2+m*(g)*Jp3;

%G=G1.';

G=[0;0;0];

== matlab function CusakisME4901/Torque Control/H Matrix ==
  data: H output; qqd input; l parameter; m parameter
function H = fcn(qqd,l,m)

q=[qqd(7); qqd(8); qqd(9)];
I=(1/12)*m*(l^2); 
%Hand derivation of the Jacobians for the three links
Jp1=[-(l/2)*sin(q(1)) 0 0; (l/2)*cos(q(1)) 0 0; 0 0 0];
Jo1=[0 0 0; 0 0 0; 1 0 0];

Jp2=[-l*sin(q(1))-(l/2)*sin(q(1)+q(2)) -(l/2)*sin(q(1)+q(2)) 0 ;    l*cos(q(1))+(l/2)*cos(q(1)+q(2)) (l/2)*cos(q(1)+q(2)) 0; 0 0 0];
Jo2=[0 0 0; 0 0 0; 1 1 0];

Jp3=[-l*sin(q(1))-l*sin(q(1)+q(2))-(l/2)*sin(q(1)+q(2)+q(3)) -l*sin(q(1)+q(2))-(l/2)*sin(q(1)+q(2)+q(3)) -(l/2)*sin(q(1)+q(2)+q(3)); l*cos(q(1))+(l)*cos(q(1)+q(2))+(l/2)*cos(q(1)+q(2)+q(3)) l*cos(q(1)+q(2))+(l/2)*cos(q(1)+q(2)+q(3)) (l/2)*cos(q(1)+q(2)+q(3)); 0 0 0];
Jo3=[0 0 0; 0 0 0; 1 1 1];

%%%%%%%%%%%%%%%%%%%%%%%%%%%%%%%%%%%%%%%%%%%%%%%%%%%%%%%%%%%%%%%%%%%%%%%%%
% %Inertia Matrix H
H1=(m*(Jp1')*Jp1)+(Jo1'*I*Jo1); %should be Hermitian? ???????????    
H2=(m*(Jp2')*Jp2)+(Jo2'*I*Jo2);
H3=(m*(Jp3')*Jp3)+(Jo3'*I*Jo3);
%Total Inertia Matrix
H=H1+H2+H3;

== matlab function CusakisME4901/Dynamics Block/H Matrix ==
  data: H output; qqd input; l parameter; mn parameter
function H = fcn(qqd,l,mn)

q=[qqd(7) qqd(8) qqd(9)];
I=(1/12)*mn*(l^2); 
%Hand derivation of the Jacobians for the three links
Jp1=[-(l/2)*sin(q(1)) 0 0; (l/2)*cos(q(1)) 0 0; 0 0 0];
Jo1=[0 0 0; 0 0 0; 1 0 0];

Jp2=[-l*sin(q(1))-(l/2)*sin(q(1)+q(2)) -(l/2)*sin(q(1)+q(2)) 0 ;    l*cos(q(1))+(l/2)*cos(q(1)+q(2)) (l/2)*cos(q(1)+q(2)) 0; 0 0 0];
Jo2=[0 0 0; 0 0 0; 1 1 0];

Jp3=[-l*sin(q(1))-l*sin(q(1)+q(2))-(l/2)*sin(q(1)+q(2)+q(3)) -l*sin(q(1)+q(2))-(l/2)*sin(q(1)+q(2)+q(3)) -(l/2)*sin(q(1)+q(2)+q(3)); l*cos(q(1))+(l)*cos(q(1)+q(2))+(l/2)*cos(q(1)+q(2)+q(3)) l*cos(q(1)+q(2))+(l/2)*cos(q(1)+q(2)+q(3)) (l/2)*cos(q(1)+q(2)+q(3)); 0 0 0];
Jo3=[0 0 0; 0 0 0; 1 1 1];

%%%%%%%%%%%%%%%%%%%%%%%%%%%%%%%%%%%%%%%%%%%%%%%%%%%%%%%%%%%%%%%%%%%%%%%%%
% %Inertia Matrix H
H1=(mn*(Jp1')*Jp1)+(Jo1'*I*Jo1); %should be Hermitian? ???????????    
H2=(mn*(Jp2')*Jp2)+(Jo2'*I*Jo2);
H3=(mn*(Jp3')*Jp3)+(Jo3'*I*Jo3);
%Total Inertia Matrix
H=H1+H2+H3;

== matlab function CusakisME4901/Differential Kinematics1/Activate Mobile base/MATLAB Function ==
  data: but input; y output; bo input
function y   = fcn(but,bo)
%#codegen


b=but(3);

if b==1
if bo==0
y=1;
else
y=0;
end
else
if bo==1
y=1;
else
y=0;
end
end
